simulink model "Hydraulic_Lab_BD"  (R2023b)
settings: Solver=VariableStepAuto  StartTime=0.0  StopTime=50  RelTol=1e-9
undefined symbols (not defined in the file or in its folder): A, b, beta_Vt, Ka, Kce, Kcmp, Kd, Ki, Kp, Kpot, Kq, m, st
libraries: simulink x2
settings Model: Creator=julia  LastModifiedBy=Aiden
settings SolverCC: MaxConsecutiveMinStep=5

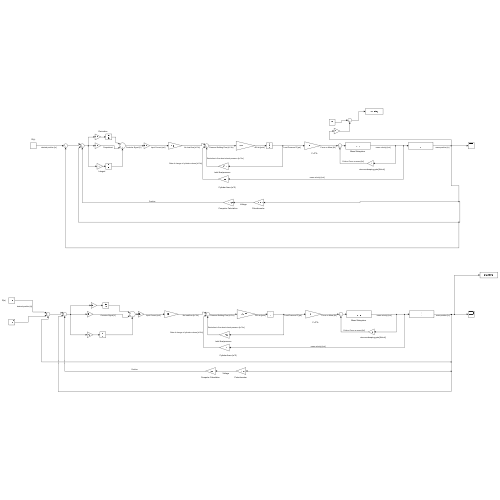
[thumbnail: Simulink's stored preview of the top-level diagram]
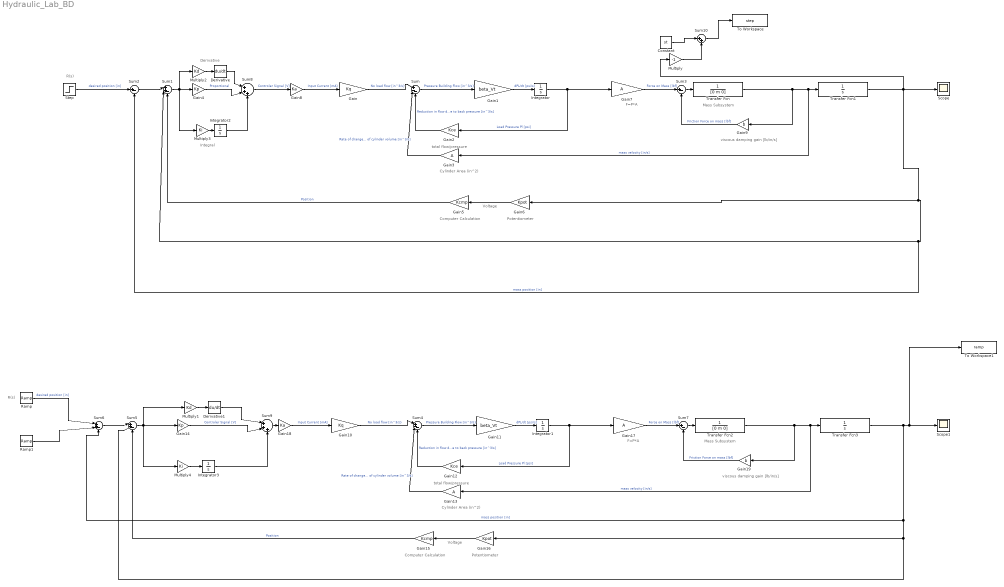
== system Hydraulic_Lab_BD ==
  note: Mass Subsystem
  note: F=P*A
  note: viscous damping gain [lb/in/s]
  note: Voltage
  note: Cylinder Area (in^2)
  note: Potentiometer
  note: Computer Calculation
  note: total flow/pressure
  note: R(s)
  note: Integral
  note: Derivative
  note: Potentiometer
  note: F=P*A
  note: Voltage
  note: Computer Calculation
  note: R(s)
  note: total flow/pressure
  note: viscous damping gain [lb/in/s]
  note: Cylinder Area (in^2)
  note: Mass Subsystem
  Constant : Constant  Value=st
  Derivative : Derivative
  Derivative1 : Derivative
  Gain : Gain  Gain=Kq
  Gain1 : Gain  Gain=beta_Vt
  Gain10 : Gain  Gain=Kq
  Gain11 : Gain  Gain=beta_Vt
  Gain12 : Gain  Gain=Kce
  Gain{3,7,13,17} (4 alike) : Gain  Gain=A
  Gain14 : Gain  Gain=Kp
  Gain15 : Gain  Gain=Kcmp
  Gain16 : Gain  Gain=Kpot
  Gain18 : Gain  Gain=Ka
  Gain19 : Gain  Gain=b
  Gain2 : Gain  Gain=Kce
  Gain4 : Gain  Gain=Kp
  Gain5 : Gain  Gain=Kcmp
  Gain6 : Gain  Gain=Kpot
  Gain8 : Gain  Gain=Ka
  Gain9 : Gain  Gain=b
  Integrator{,1..3} (4 alike) : Integrator
  Multiply : Gain  Gain=-1
  Multiply1 : Gain  Gain=Kd
  Multiply2 : Gain  Gain=Kd
  Multiply3 : Gain  Gain=Ki
  Multiply4 : Gain  Gain=Ki
  Ramp : simulink/Sources/Ramp  slope=-4  start=2  InitialOutput=2
  Ramp1 : simulink/Sources/Ramp  slope=4  start=3  InitialOutput=0
  Scope : Scope
  Scope1 : Scope
  Step : Step  Time=2  After=st  SampleTime=0
  Sum : Sum  Inputs=|+--
  Sum1 : Sum  Inputs=|++-
  Sum10 : Sum  Inputs=|++
  Sum2 : Sum  Inputs=|+-
  Sum3 : Sum  Inputs=|+-
  Sum4 : Sum  Inputs=|+--
  Sum5 : Sum  Inputs=|++-
  Sum6 : Sum  Inputs=|++-
  Sum7 : Sum  Inputs=|+-
  Sum8 : Sum  Inputs=|+++
  Sum9 : Sum  Inputs=|+++
  To Workspace : ToWorkspace  VariableName=step  SampleTime=-1
  To Workspace1 : ToWorkspace  VariableName=ramp  SampleTime=-1
  Transfer Fcn : TransferFcn  Denominator=[0 m 0]
  Transfer Fcn1 : TransferFcn  Denominator=[0 1 0]
  Transfer Fcn2 : TransferFcn  Denominator=[0 m 0]
  Transfer Fcn3 : TransferFcn  Denominator=[0 1 0]
  wires:
  Gain10/1 -> Sum4/1  "No load flow [in^3/s}"
  Ramp/1 -> Sum6/1  "desired position [in]"
  Gain15/1 -> Sum5/3  "Position"
  Sum5/1 -> Multiply1/1, Multiply4/1, Gain14/1
  Multiply4/1 -> Integrator3/1
  Gain17/1 -> Sum7/1  "Force on Mass [lbf]"
  Gain12/1 -> Sum4/3  "Reduction in flow due to back pressure [in^3/s]"
  Multiply1/1 -> Derivative1/1
  Sum4/1 -> Gain11/1  "Pressure Building Flow [in^3/s}"
  Sum9/1 -> Gain18/1
  Integrator3/1 -> Sum9/3
  Gain11/1 -> Integrator1/1  "dPL/dt [psi/s]"
  Transfer Fcn3/1 -> To Workspace1/1, Scope1/1, Sum6/3, Sum5/2, Gain16/1  "mass position [in]"
  Gain13/1 -> Sum4/2  "Rate of change of cylinder volume [in^3/s]"
  Gain18/1 -> Gain10/1  "Input Current [mA]"
  Gain19/1 -> Sum7/2  "Friction Force on mass [lbf]"
  Gain16/1 -> Gain15/1
  Transfer Fcn2/1 -> Gain13/1, Transfer Fcn3/1, Gain19/1  "mass velocity [in/s]"
  Integrator1/1 -> Gain12/1, Gain17/1  "Load Pressure Pl [psi]"
  Sum6/1 -> Sum5/1
  Ramp1/1 -> Sum6/2
  Derivative1/1 -> Sum9/1
  Sum7/1 -> Transfer Fcn2/1
  Gain14/1 -> Sum9/2  "Controler Signal [V]"
  Sum10/1 -> To Workspace/1
  Constant/1 -> Sum10/1
  Multiply3/1 -> Integrator2/1
  Transfer Fcn1/1 -> Multiply/1, Sum2/2, Sum1/2, Gain6/1, Scope/1  "mass position [in]"
  Derivative/1 -> Sum8/1
  Sum3/1 -> Transfer Fcn/1
  Gain9/1 -> Sum3/2  "Friction Force on mass [lbf]"
  Sum2/1 -> Sum1/1
  Gain2/1 -> Sum/3  "Reduction in flow due to back pressure [in^3/s]"
  Multiply/1 -> Sum10/2
  Gain4/1 -> Sum8/2  "Proportional"
  Sum/1 -> Gain1/1  "Pressure Building Flow [in^3/s}"
  Gain8/1 -> Gain/1  "Input Current [mA]"
  Integrator2/1 -> Sum8/3
  Transfer Fcn/1 -> Gain3/1, Transfer Fcn1/1, Gain9/1  "mass velocity [in/s]"
  Multiply2/1 -> Derivative/1
  Step/1 -> Sum2/1  "desired position [in]"
  Gain7/1 -> Sum3/1  "Force on Mass [lbf]"
  Gain6/1 -> Gain5/1
  Gain5/1 -> Sum1/3  "Position"
  Sum1/1 -> Multiply2/1, Multiply3/1, Gain4/1
  Gain/1 -> Sum/1  "No load flow [in^3/s}"
  Sum8/1 -> Gain8/1  "Controler Signal [V]"
  Gain1/1 -> Integrator/1  "dPL/dt [psi/s]"
  Gain3/1 -> Sum/2  "Rate of change of cylinder volume [in^3/s]"
  Integrator/1 -> Gain2/1, Gain7/1  "Load Pressure Pl [psi]"
